simulink model "robot_traj"  (R2021b)
settings: Solver=VariableStepAuto  StartTime=0.0  StopTime=76  RelTol=1e-3
libraries: roblocks x17, simulink x6
settings Model: Creator=sam  LastModifiedBy=sam

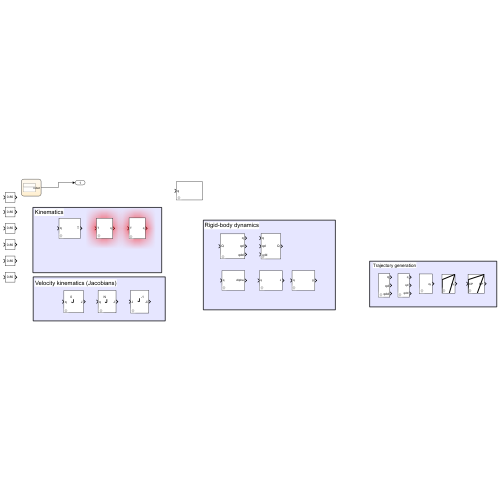
[thumbnail: Simulink's stored preview of the top-level diagram]
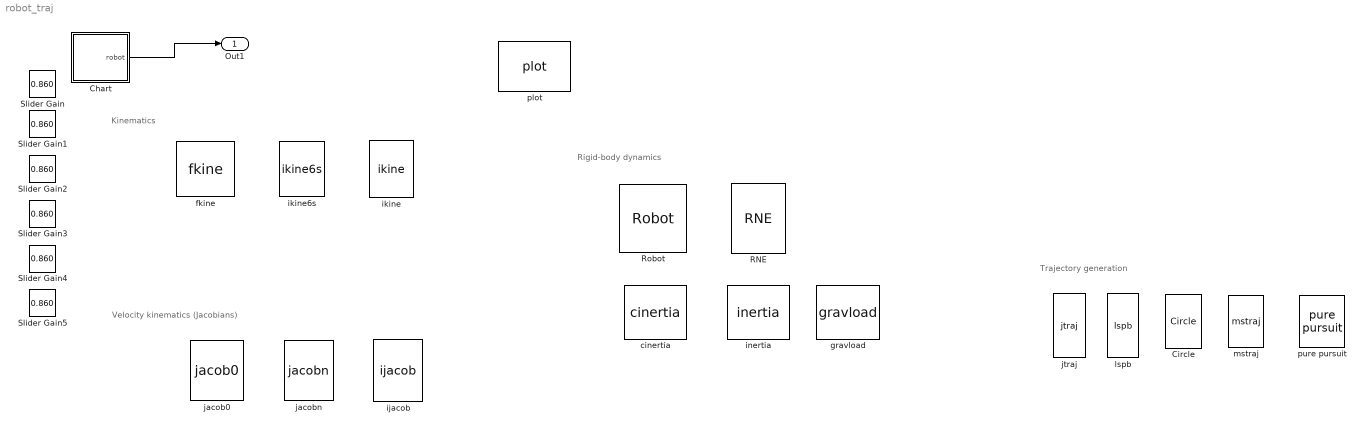
== system robot_traj ==
  note: Rigid-body dynamics
  note: Velocity kinematics (Jacobians)
  note: Kinematics
  note: Trajectory generation
  Chart : Stateflow chart  TreatAsAtomicUnit=on
  Circle : roblocks/Toolbox/Circle  radius=1  freq=0.2
  RNE : roblocks/Arm/RNE  robot=robot  grav=[0 0 9.81]
  Robot : roblocks/Arm/Robot  robot=robot  q0=[0 0 0 0 0 0]
  Slider Gain{,1..5} (6 alike) : simulink/Math Operations/Slider Gain  gain=0.860  low=0  high=2
  cinertia : roblocks/Arm/cinertia  robot=0
  fkine : roblocks/Arm/fkine  robot=robot
  gravload : roblocks/Arm/gravload  robot=0
  ijacob : roblocks/Arm/ijacob
  ikine : roblocks/Arm/ikine  robot=p560  q0=qz  M=[1 1 1 1 1 1]  pinv=off  options={}
  ikine6s : roblocks/Arm/ikine6s  robot=p560  conf='luf'
  inertia : roblocks/Arm/inertia  robot=0
  "jacob0 " : roblocks/Arm/jacob0   robot=robot
  jacobn : roblocks/Arm/jacobn  robot=robot
  jtraj : roblocks/Toolbox/jtraj  q0=[0 0 0 0 0 0]  qf=[pi/4 pi/2 -pi/2 0 0 0]  tmax=10  ts=0.02
  lspb : roblocks/Toolbox/lspb  q0=0  qf=0  tmax=0
  mstraj : roblocks/Toolbox/mstraj  path=|  vaxis=[2.5 2.5]  tseg=[]  dt=0.1  tacc=0  setsimtime=on
      | [  10 10;
      |   10 60;
      |   80 80;
      |   50 10 ]
  plot : roblocks/Arm/plot  robot=tecoarm  fps=5  holdplot=on
  pure pursuit : roblocks/Toolbox/pure pursuit  path=|  vaxis=[2.5 2.5]  tseg=[]  dt=0.1  tacc=0  R=5
      | [  10 10;
      |   10 60;
      |   80 80;
      |   50 10 ]
  Out1 : Outport
  wires:
  Chart/1(robot) -> Out1/1

== matlab function robot_traj/Chart ==
  data: tecoarm function_output; robot output
function tecoarm = robot_arm_init()
%%%%%%%%%%%%%%%%%%%%%%%%
%% 建立機器人模型
        % theta    d        a        alpha     offset
        %L1 = Link([0 0.2 1 pi/4 0],'standard'); %標準模式 L1 = Link([0 0.2 1
        %pi/4 0],'modify'); %改進模式
% mass = [3.7000, 8.3930, 2.33, 1.2190, 1.2190, 0.1897];

% center_of_mass = [
%         0,-0.02561, 0.00193
%         0.2125, 0, 0.11336
%         0.15, 0, 0.0265
%         0, -0.0018, 0.01634
%         0, -0.0018, 0.01634
%         0, 0, -0.001159];
%不寫默認標準模式 % robot length values (metres)
L1=Link([0       0.08916    0        pi/2      0     ],'standard'); 
L2=Link([0       0        0.425     0         0     ],'standard');
L3=Link([0       0        0.39225   0         0     ],'standard');
L4=Link([0       0.10915   0        pi/2      0     ],'standard');
L5=Link([0       0.09456    0        -pi/2     0     ],'standard');
L6=Link([0       0.0823     0        0         0     ],'standard');
tecoarm = SerialLink([L1 L2 L3 L4 L5 L6],'name','tecoarm')%連接連桿，機器人命名
